simulink model "Lab1A_C4"  (R2019b)
settings: Solver=ode4  StartTime=0.0  StopTime=4  FixedStep=1e-2  RelTol=1e-3
settings Model: Creator=sinow  LastModifiedBy=sinow

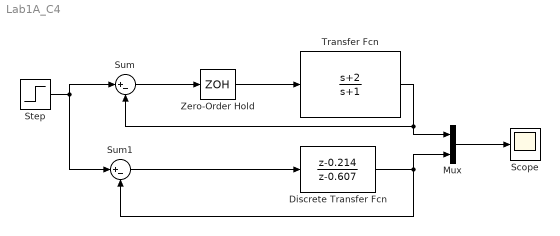
== system Lab1A_C4 ==
  Discrete Transfer Fcn : DiscreteTransferFcn  Numerator=[1 -0.214]  Denominator=[1 -0.607]  SampleTime=0.5
  Mux : Mux  Inputs=2
  Scope : Scope
  Step : Step  Time=0  SampleTime=0
  Sum : Sum  Inputs=|+-
  Sum1 : Sum  Inputs=|+-
  Transfer Fcn : TransferFcn  Numerator=[1 2]  Denominator=[1 1]
  Zero-Order Hold : ZeroOrderHold  SampleTime=0.5
  wires:
  Step/1 -> Sum1/1, Sum/1
  Sum/1 -> Zero-Order Hold/1
  Zero-Order Hold/1 -> Transfer Fcn/1
  Transfer Fcn/1 -> Sum/2, Mux/1
  Discrete Transfer Fcn/1 -> Sum1/2, Mux/2
  Mux/1 -> Scope/1
  Sum1/1 -> Discrete Transfer Fcn/1
